simulink model "Aeropendulum"  (R2017b)
settings: Solver=VariableStepAuto  StartTime=0.0  StopTime=30  RelTol=1e-3
values from neighbouring files (symbols this model uses):
  c = 0.01    [Main.m]
  d = 0.023    [Main.m]
  g = 9.80665    [Main.m]
  J = 0.0090    (= 0.009)    [Main.m]
  L = 0.495    [Main.m]
  m = 0.43    [Main.m]
libraries: simulink_extras x6, fuzblock x4, neural x1, simulink x1
settings Model: Creator=emerrf  LastModifiedBy=Josep Famadas
settings SolverCC: AlgebraicLoopSolver=LineSearch

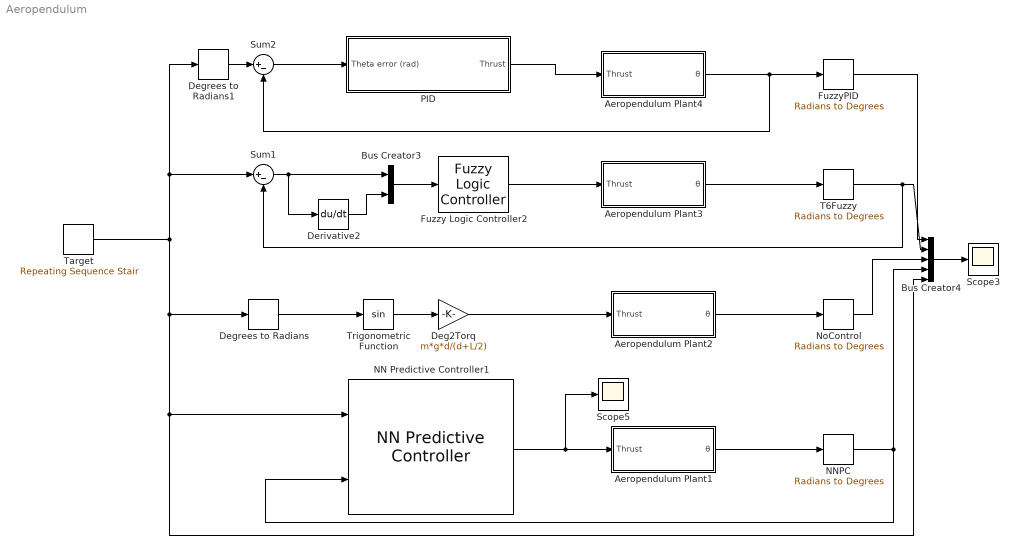
== system Aeropendulum ==
  Aeropendulum Plant1 : Subsystem
  Aeropendulum Plant2 : Subsystem
  Aeropendulum Plant3 : Subsystem
  Aeropendulum Plant4 : Subsystem
  Bus Creator3 : BusCreator  Inputs=2
  Bus Creator4 : BusCreator  Inputs=5
  Deg2Torq : Gain  Gain=m*g*d/(d+L/2)
  Degrees to Radians : simulink_extras/Transformations/Degrees to Radians
  Degrees to Radians1 : simulink_extras/Transformations/Degrees to Radians
  Derivative2 : Derivative
  Fuzzy Logic Controller2 : fuzblock/Fuzzy Logic  Controller  FIS='task6_fuzzy_controller.fis'  OutputSampleNumber=101  DataType=double  FuzzifiedInputs=off  RuleFiringStrengths=off  RuleOutputs=off  AggregatedOutputs=off  SimulateUsing=Interpreted execution
  FuzzyPID : simulink_extras/Transformations/Radians to Degrees
  NN Predictive Controller1 : neural/Control Systems/NN Predictive Controller  epochs=20000  minp=-0.2101672440322849833  maxp=0.24372391469033249933  mint=-88.833199595274393801  maxt=0.24372391469033249933  Normalize=0  IW=[-0.23857564621853699638;1.5584676525855500895;0.012247948624780988919;0.042946463219871458539;-8.0651579612770110117;5.9245348142503351241;0.018743364866522425199]  LW1_2=[4.7631167282761062154 5.9490506053056275704 7.0754379408506284932;-8.462556833091072761 1.0083684270652435444 2.1867613296671861711;0.04319828463912826072 -0.042876868543869989248 0.014295001166202789267;0.022782826173060086172 -0.011733986317698584523 0.00034820361933919321195;3.9322093856642825749 -7.8246745772169310484 2.0797518098966705224;-9.5002396516435183571 3.0077343931861060256 1.2003153506926655947;0.028171729089119947054 -0.024083465139735731747 0.0067568840575017493494]  LW2_1=[5.8018317869437285143e-06 4.4651976365140937375 42.817885186759681915 46.386912030301218124 0.0013850830984490675353 -4.4656667947412458375 70.035253742111549968]  B1=[-3.7357431340586391144;5.6975612807707847196;1.3609807721418838433;0.13257921402934286226;5.3959286772480430372;5.6950899253017972512;-0.99930689639239511646]  B2=9.6684672643688838178  max_i_int=15  min_i_int=5  limit_output=0  max_output=Inf  min_output=-Inf  Use_Previous_Weights=1  N2=10  Nu=5  Ts=0.05  rho=0.05  alpha=0.001  csrchfun=csrchbac  maxiter=2  S1=7  Ni=1  Nj=3  sim_file=aeropendulum_model  trainfun=trainlm  Use_validation=1  Use_Testing=1  max_i=0.246  min_i=-0.246  sam_training=10000
      settings: SourceProductName=Neural Network Toolbox  SourceProductBaseCode=NN
  NNPC : simulink_extras/Transformations/Radians to Degrees
  NoControl : simulink_extras/Transformations/Radians to Degrees
  PID : Subsystem
  Scope3 : Scope
  Scope5 : Scope
  Sum1 : Sum  Inputs=|+-
  Sum2 : Sum  Inputs=|+-
  T6Fuzzy : simulink_extras/Transformations/Radians to Degrees
  Target : simulink/Sources/Repeating Sequence Stair  OutValues=[20 25 10 15].'  tsamp=5  OutMin=[]  OutMax=[]  OutDataTypeStr=double  OutputDataTypeScalingMode=double  OutDataType=fixdt(0,8)  ConRadixGroup=Best Precision: Vector-wise  OutScaling=2^-12
  Trigonometric Function : Trigonometry
  wires:
  Fuzzy Logic Controller2/1 -> Aeropendulum Plant3/1(Thrust)
  NoControl/1 -> Bus Creator4/3
  Sum1/1 -> Derivative2/1, Bus Creator3/1
  T6Fuzzy/1 -> Bus Creator4/2, Sum1/2
  Derivative2/1 -> Bus Creator3/2
  Bus Creator4/1 -> Scope3/1
  Bus Creator3/1 -> Fuzzy Logic Controller2/1
  NNPC/1 -> NN Predictive Controller1/2, Bus Creator4/4
  Aeropendulum Plant3/1(θ) -> T6Fuzzy/1
  Aeropendulum Plant2/1(θ) -> NoControl/1
  NN Predictive Controller1/1 -> Scope5/1, Aeropendulum Plant1/1(Thrust)
  Aeropendulum Plant1/1(θ) -> NNPC/1
  Trigonometric Function/1 -> Deg2Torq/1
  Deg2Torq/1 -> Aeropendulum Plant2/1(Thrust)
  Degrees to Radians/1 -> Trigonometric Function/1
  Target/1 -> NN Predictive Controller1/1, Bus Creator4/5, Degrees to Radians/1, Degrees to Radians1/1, Sum1/1
  Aeropendulum Plant4/1(θ) -> Sum2/2, FuzzyPID/1
  PID/1(Thrust) -> Aeropendulum Plant4/1(Thrust)
  Sum2/1 -> PID/1(Theta error (rad))
  Degrees to Radians1/1 -> Sum2/1
  FuzzyPID/1 -> Bus Creator4/1

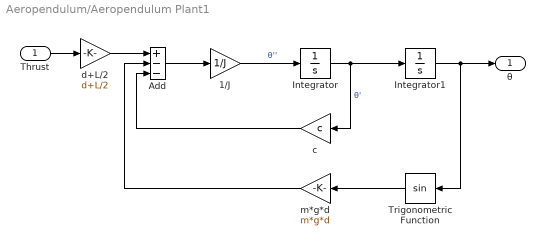
== system Aeropendulum/Aeropendulum Plant1 ==
  Thrust : Inport
  1/J : Gain  Gain=1/J
  Add : Sum  Inputs=+--
  Integrator : Integrator
  Integrator1 : Integrator
  Trigonometric Function : Trigonometry
  c : Gain  Gain=c
  d+L/2 : Gain  Gain=d+L/2
  m*g*d : Gain  Gain=m*g*d
  θ : Outport
  wires:
  Thrust/1 -> d+L/2/1
  Add/1 -> 1/J/1
  1/J/1 -> Integrator/1  "θ''"
  Integrator/1 -> c/1, Integrator1/1  "θ'"
  Integrator1/1 -> Trigonometric Function/1, θ/1
  Trigonometric Function/1 -> m*g*d/1
  m*g*d/1 -> Add/2
  c/1 -> Add/3
  d+L/2/1 -> Add/1

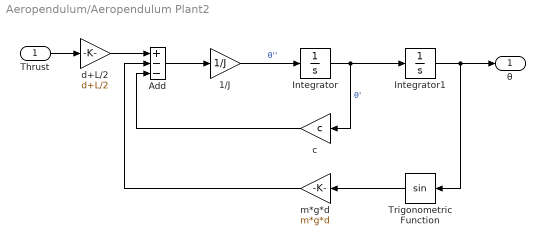
== system Aeropendulum/Aeropendulum Plant2 ==
  Thrust : Inport
  1/J : Gain  Gain=1/J
  Add : Sum  Inputs=+--
  Integrator : Integrator
  Integrator1 : Integrator
  Trigonometric Function : Trigonometry
  c : Gain  Gain=c
  d+L/2 : Gain  Gain=d+L/2
  m*g*d : Gain  Gain=m*g*d
  θ : Outport
  wires:
  Thrust/1 -> d+L/2/1
  Add/1 -> 1/J/1
  1/J/1 -> Integrator/1  "θ''"
  Integrator/1 -> c/1, Integrator1/1  "θ'"
  Integrator1/1 -> Trigonometric Function/1, θ/1
  Trigonometric Function/1 -> m*g*d/1
  m*g*d/1 -> Add/2
  c/1 -> Add/3
  d+L/2/1 -> Add/1

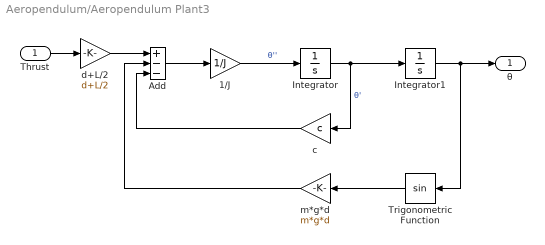
== system Aeropendulum/Aeropendulum Plant3 ==
  Thrust : Inport
  1/J : Gain  Gain=1/J
  Add : Sum  Inputs=+--
  Integrator : Integrator
  Integrator1 : Integrator
  Trigonometric Function : Trigonometry
  c : Gain  Gain=c
  d+L/2 : Gain  Gain=d+L/2
  m*g*d : Gain  Gain=m*g*d
  θ : Outport
  wires:
  Thrust/1 -> d+L/2/1
  Add/1 -> 1/J/1
  1/J/1 -> Integrator/1  "θ''"
  Integrator/1 -> c/1, Integrator1/1  "θ'"
  Integrator1/1 -> Trigonometric Function/1, θ/1
  Trigonometric Function/1 -> m*g*d/1
  m*g*d/1 -> Add/2
  c/1 -> Add/3
  d+L/2/1 -> Add/1

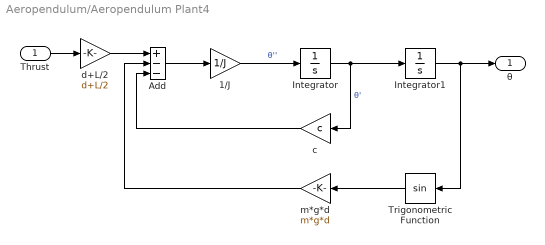
== system Aeropendulum/Aeropendulum Plant4 ==
  Thrust : Inport
  1/J : Gain  Gain=1/J
  Add : Sum  Inputs=+--
  Integrator : Integrator
  Integrator1 : Integrator
  Trigonometric Function : Trigonometry
  c : Gain  Gain=c
  d+L/2 : Gain  Gain=d+L/2
  m*g*d : Gain  Gain=m*g*d
  θ : Outport
  wires:
  Thrust/1 -> d+L/2/1
  Add/1 -> 1/J/1
  1/J/1 -> Integrator/1  "θ''"
  Integrator/1 -> c/1, Integrator1/1  "θ'"
  Integrator1/1 -> Trigonometric Function/1, θ/1
  Trigonometric Function/1 -> m*g*d/1
  m*g*d/1 -> Add/2
  c/1 -> Add/3
  d+L/2/1 -> Add/1

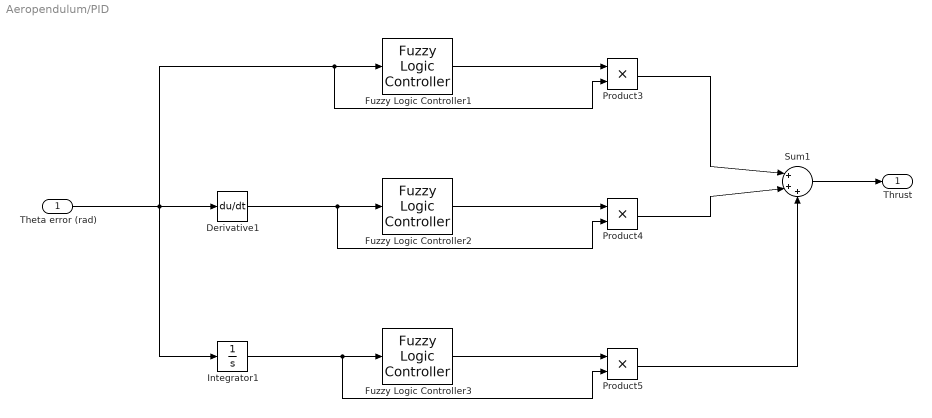
== system Aeropendulum/PID ==
  Theta error (rad) : Inport
  Derivative1 : Derivative
  Fuzzy Logic Controller1 : fuzblock/Fuzzy Logic  Controller  FIS='task6_fuzzy_controllerPID.fis'  OutputSampleNumber=101  DataType=double  FuzzifiedInputs=off  RuleFiringStrengths=off  RuleOutputs=off  AggregatedOutputs=off  SimulateUsing=Interpreted execution
  Fuzzy Logic Controller2 : fuzblock/Fuzzy Logic  Controller  FIS='task6_fuzzy_controllerPID.fis'  OutputSampleNumber=101  DataType=double  FuzzifiedInputs=off  RuleFiringStrengths=off  RuleOutputs=off  AggregatedOutputs=off  SimulateUsing=Interpreted execution
  Fuzzy Logic Controller3 : fuzblock/Fuzzy Logic  Controller  FIS='task6_fuzzy_controllerPID.fis'  OutputSampleNumber=101  DataType=double  FuzzifiedInputs=off  RuleFiringStrengths=off  RuleOutputs=off  AggregatedOutputs=off  SimulateUsing=Interpreted execution
  Integrator1 : Integrator
  Product3 : Product
  Product4 : Product
  Product5 : Product
  Sum1 : Sum  Inputs=|+++
  Thrust : Outport
  wires:
  Integrator1/1 -> Product5/2, Fuzzy Logic Controller3/1
  Product5/1 -> Sum1/3
  Fuzzy Logic Controller1/1 -> Product3/1
  Product4/1 -> Sum1/2
  Product3/1 -> Sum1/1
  Fuzzy Logic Controller3/1 -> Product5/1
  Fuzzy Logic Controller2/1 -> Product4/1
  Sum1/1 -> Thrust/1
  Theta error (rad)/1 -> Product3/2, Fuzzy Logic Controller1/1, Integrator1/1, Derivative1/1
  Derivative1/1 -> Product4/2, Fuzzy Logic Controller2/1
